simulink subsystem "MR_MainRotorForcesMoments"  (R2025a)
settings: Solver=VariableStepAuto  StartTime=0.0  StopTime=20  RelTol=1e-3
undefined symbols (not defined in the file): MR_BEDistFromEffSta_A, MR_BladeFlapInertia_P, MR_RotationMatrix_A, MR_RotorRadius_P, MR_TranslationMatrix_A
libraries: simulink_extras x4
settings Model: DataDictionary=MainRotor.sldd  EnableAccessToBaseWorkspace=off  DefaultTestHarness=MR_MainRotorForcesMoments_Harness_v1  Creator=Admin  LastModifiedBy=tunglt60

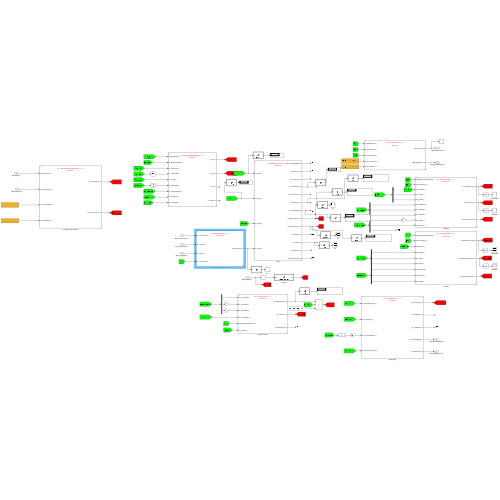
[thumbnail: Simulink's stored preview of the top-level diagram]
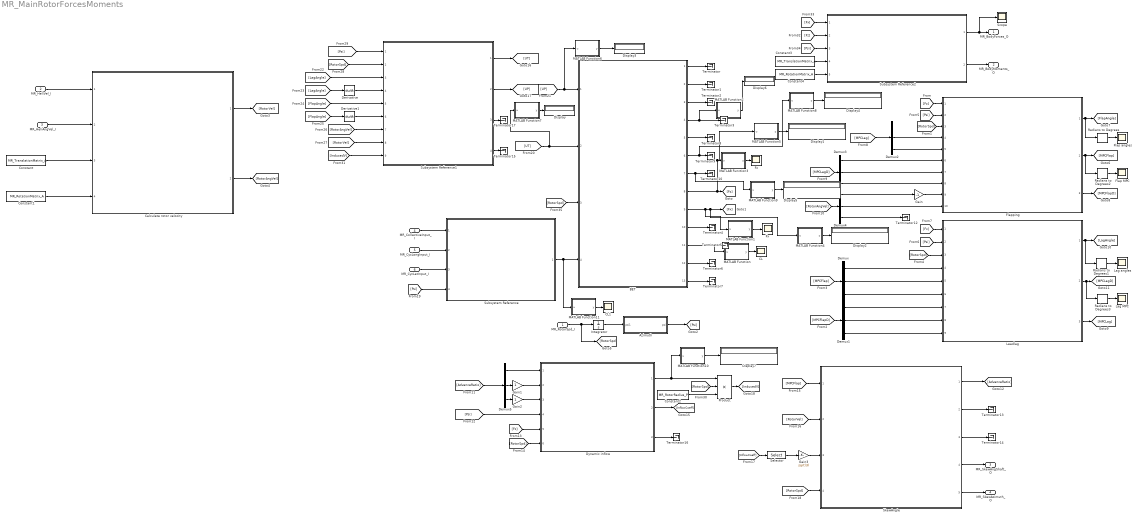
== system MR_MainRotorForcesMoments ==
  MR_RotorSpd_I : Inport
  MR_HeliVel_I : Inport  Port=2
  MR_HeliAngVel_I : Inport  Port=3
  MR_CollectiveInput_I : Inport  Port=4
  MR_CycLongInput_I : Inport  Port=5
  MR_CycLatInput_I : Inport  Port=6
  Azimuth : MATLAB Function  TreatAsAtomicUnit=on
  BET : Subsystem  ReferencedSubsystem=RT_BladeElementForces_v1_2  RT_Weight=MR_Weight_P  RT_AirDensity=MR_AirDensity_P  RT_RotorRadius=MR_RotorRadius_P  RT_NondimRadialDisRef=MR_NondimRadialDisRef_P  RT_BEDistFromEffSta=MR_BEDistFromEffSta_A  RT_SonicVel=MR_SonicVel_P  RT_SigmaAvgUH60=MR_SigmaAvgUH60_P  RT_NumberOfBlades=MR_NumberOfBlades_P  RT_TaperedRatio=MR_TaperedRatio_P
      settings: PermitHierarchicalResolution=None
  CL : Scope
      settings: ActiveDisplayYMinimum=44.632677219463247  ActiveDisplayYMaximum=47.250297558148787  DataLoggingVariableName=ScopeData5
  CL1 : Scope
      settings: ActiveDisplayYMinimum=0.59813170079773181  ActiveDisplayYMaximum=0.79813170079773177  DataLoggingVariableName=ScopeData10
  Calculate rotor velocity : Subsystem  ReferencedSubsystem=RT_HubLinearAndAngularVelocity_v1_1
      settings: PermitHierarchicalResolution=None
  Constant : Constant  Value=MR_TranslationMatrix_A
  Constant1 : Constant  Value=MR_RotationMatrix_A
  Constant2 : Constant  Value=MR_RotorRadius_P
  Constant3 : Constant  Value=MR_TranslationMatrix_A
  Constant4 : Constant  Value=MR_RotationMatrix_A
  Demux{,1..5} (6 alike) : Demux  Outputs=3
  Derivative : Derivative
  Derivative1 : Derivative
  Display{,1..7} (8 alike) : Display
  Dynamic inflow : Subsystem  ReferencedSubsystem=RT_DynamicInflow_V1_2  RT_BEDistFromEffSta=MR_BEDistFromEffSta_A  RT_AirDensity=MR_AirDensity_P  RT_RotorRadius=MR_RotorRadius_P
  Flap MPC : Scope
      settings: ActiveDisplayYMinimum=-75.476403877152109  ActiveDisplayYMaximum=118.89472721519165  DataLoggingVariableName=ScopeData4
  Flap angles : Scope
      settings: ActiveDisplayYMinimum=-1.4856198695096292  ActiveDisplayYMaximum=13.370578825586666  DataLoggingVariableName=ScopeData8
  Flapping : Subsystem  ReferencedSubsystem=RT_FlappingDynamic_v1_2  RT_BEDistFromEffSta=MR_BEDistFromEffSta_A  RT_RotorRadius=MR_RotorRadius_P  RT_BladeFlapInertia=MR_BladeFlapInertia_P*2  RT_BEMassFromHinge=MR_BEMassFromHinge_A  RT_BEDistFromHinge=MR_BEDistFromHinge_A  RT_HingeFlapPos=MR_HingeFlapPos_P
      settings: PermitHierarchicalResolution=None
  Fx : Scope
      settings: ActiveDisplayYMinimum=-148.02372012161376  ActiveDisplayYMaximum=1332.213481094524  DataLoggingVariableName=ScopeData7
  Fz : Scope
      settings: ActiveDisplayYMinimum=-361.43274494516839  ActiveDisplayYMaximum=97.915180558424424  DataLoggingVariableName=ScopeData6
  Gain : Gain  Gain=-1
  Gain1 : Gain
  Gain2 : Gain
  Gain3 : Gain  Gain=sqrt(3)
  Integrator : Integrator
  Lag MPC : Scope
      settings: ActiveDisplayYMinimum=-20550.82418968204  ActiveDisplayYMaximum=3886.6217076516573  DataLoggingVariableName=ScopeData9
  Lag angles : Scope
      settings: ActiveDisplayYMinimum=-1.032742411790134  ActiveDisplayYMaximum=9.29468170611121  DataLoggingVariableName=ScopeData3
  Leadlag : Subsystem  ReferencedSubsystem=RT_LeadLagDynamic_v1_2  RT_BEDistFromEffSta=MR_BEDistFromEffSta_A  RT_RotorRadius=MR_RotorRadius_P  RT_BEMassFrHingeLead=MR_BEMassFrHingeLead_A  RT_BEDistFrHingeLead=MR_BEDistFrHingeLead_A  RT_HingeLeadPos=MR_HingeLeadPos_P  RT_BladeLeadInertia=MR_BladeLeadInertia_P
      settings: PermitHierarchicalResolution=None
  MATLAB Function : MATLAB Function  TreatAsAtomicUnit=on
  MATLAB Function1 : MATLAB Function  TreatAsAtomicUnit=on
  MATLAB Function10 : MATLAB Function  TreatAsAtomicUnit=on
  MATLAB Function11 : MATLAB Function  TreatAsAtomicUnit=on
  MATLAB Function2 : MATLAB Function  TreatAsAtomicUnit=on
  MATLAB Function3 : MATLAB Function  TreatAsAtomicUnit=on
  MATLAB Function4 : MATLAB Function  TreatAsAtomicUnit=on
  MATLAB Function5 : MATLAB Function  TreatAsAtomicUnit=on
  MATLAB Function6 : MATLAB Function  TreatAsAtomicUnit=on
  MATLAB Function7 : MATLAB Function  TreatAsAtomicUnit=on
  MATLAB Function8 : MATLAB Function  TreatAsAtomicUnit=on
  MATLAB Function9 : MATLAB Function  TreatAsAtomicUnit=on
  Product : Product  Inputs=3
  Radians to Degrees{,1..3} (4 alike) : simulink_extras/Transformations/Radians to Degrees
  Scope : Scope
      settings: ActiveDisplayYMinimum=-141063.76400724504  ActiveDisplayYMaximum=27745.518592348737  DataLoggingVariableName=ScopeData11
  Selector : Selector  InputPortWidth=3  IndexOptions=Index vector (dialog)  Indices=1  OutputSizes=1
  SkewAngle : Subsystem  ReferencedSubsystem=RT_SkewCalculation_V1_2  RT_RotorRadius=MR_RotorRadius_P
  Subsystem Reference : Subsystem  ReferencedSubsystem=RT_BladePitchAngles_v1_2
  Subsystem Reference1 : Subsystem  ReferencedSubsystem=RT_RelativeWindOnAllBlade_v1_2  RT_BladeSegment=MR_NumberOfSegments_P  RT_BEDistFromEffSta=MR_BEDistFromEffSta_A*MR_RotorRadius_P
      settings: PermitHierarchicalResolution=None
  Subsystem Reference2 : Subsystem  ReferencedSubsystem=RT_ForcesMoments_v1_2  RT_BEDistanceToEffSta=MR_BEDistFromEffSta_A
      settings: PermitHierarchicalResolution=None
  Terminator{,1..10,12..17} (17 alike) : Terminator
  MR_BodyForces_O : Outport
  MR_BodyMoments_O : Outport  Port=2
  MR_SkewAngShaft_O : Outport  Port=3
  MR_SkewAzimuth_O : Outport  Port=4
  wires:
  BET/8 -> MATLAB Function3/1(u), MATLAB Function5/1(u), [Fz]
  BET/9 -> MATLAB Function1/1(u), [Fx], MATLAB Function4/1(u)
  BET/1 -> Terminator/1
  BET/2 -> Terminator1/1
  BET/10 -> Terminator4/1
  BET/11 -> Terminator5/1, MATLAB Function/1(u)
  BET/12 -> Terminator6/1
  BET/13 -> Terminator7/1
  BET/5 -> Terminator8/1
  BET/6 -> Terminator9/1, MATLAB Function8/1(u)
  BET/3 -> Terminator2/1
  BET/4 -> MATLAB Function2/1(u), Terminator3/1
  BET/7 -> Terminator10/1, MATLAB Function9/1(u)
  Integrator/1 -> Azimuth/1(psi1)
  Azimuth/1(psi) -> [Psi]
  MR_HeliVel_I/1 -> Calculate rotor velocity/1
  Constant/1 -> Calculate rotor velocity/3
  Constant1/1 -> Calculate rotor velocity/4
  MR_HeliAngVel_I/1 -> Calculate rotor velocity/2
  Calculate rotor velocity/2 -> [RotorAngVel]
  Calculate rotor velocity/1 -> [RotorVel]
  [Fz] -> Flapping/1
  MR_RotorSpd_I/1 -> [RotorSpd], Integrator/1
  [RotorSpd] -> Flapping/3
  Flapping/3 -> [MPCFlapD]
  Flapping/1 -> Radians to Degrees/1, [FlapAngle]
  Leadlag/1 -> Radians to Degrees1/1, [LagAngle]
  Leadlag/2 -> [MPCLagD], Radians to Degrees3/1
  Leadlag/3 -> [MPCLag]
  Demux/1 -> Leadlag/4
  Demux/2 -> Leadlag/5
  Demux/3 -> Leadlag/6
  [MPCFlap] -> Demux/1
  [MPCFlapD] -> Demux1/1
  Demux1/2 -> Leadlag/8
  Demux1/1 -> Leadlag/7
  Demux1/3 -> Leadlag/9
  [RotorSpd] -> Leadlag/3
  [Psi] -> Flapping/2
  [Psi] -> Leadlag/2
  [Fx] -> Leadlag/1
  [MPCLag] -> Demux2/1
  [MPCLagD] -> Demux3/1
  Demux3/1 -> Flapping/6
  [RotorAngVel] -> Demux4/1
  Demux4/1 -> Gain/1
  Gain/1 -> Flapping/9
  Demux4/2 -> Flapping/10
  Demux4/3 -> Terminator12/1
  Demux3/2 -> Flapping/7
  Demux3/3 -> Flapping/8
  Gain1/1 -> Dynamic inflow/2
  Gain2/1 -> Dynamic inflow/3
  SkewAngle/1 -> [AdvanceRatio]
  SkewAngle/2 -> Terminator13/1
  SkewAngle/3 -> Terminator14/1
  SkewAngle/4 -> MR_SkewAngShaft_O/1
  SkewAngle/5 -> MR_SkewAzimuth_O/1
  Demux5/2 -> Gain1/1
  Demux5/3 -> Gain2/1
  Demux5/1 -> Dynamic inflow/1
  [AdvanceRatio] -> Demux5/1
  [Psi] -> Dynamic inflow/4
  [Fz] -> Dynamic inflow/5
  [RotorSpd] -> Dynamic inflow/6
  [MPCFlap] -> SkewAngle/1
  [RotorVel] -> SkewAngle/2
  Dynamic inflow/2 -> [InflowCoeff]
  Dynamic inflow/3 -> Terminator16/1
  [InflowCoeff] -> Selector/1
  Selector/1 -> Gain3/1
  Gain3/1 -> SkewAngle/3
  [RotorSpd] -> SkewAngle/4
  MR_CycLongInput_I/1 -> Subsystem Reference/2
  MR_CycLatInput_I/1 -> Subsystem Reference/3
  MR_CollectiveInput_I/1 -> Subsystem Reference/1
  [Psi] -> Subsystem Reference/4
  Subsystem Reference/1 -> BET/4, MATLAB Function11/1(u)
  Subsystem Reference1/4 -> Terminator15/1
  Subsystem Reference1/2 -> [UP]
  Subsystem Reference1/1 -> [UT]
  [UT] -> MATLAB Function7/1(u), BET/2
  [UP] -> BET/1, MATLAB Function6/1(u)
  [RotorAngVel] -> Subsystem Reference1/7
  [RotorVel] -> Subsystem Reference1/8
  [RotorSpd] -> Subsystem Reference1/2
  [Psi] -> Subsystem Reference1/1
  Dynamic inflow/1 -> Product/1, MATLAB Function10/1(u)
  Constant2/1 -> Product/3
  [RotorSpd] -> Product/2
  Product/1 -> [InducedV]
  [InducedV] -> Subsystem Reference1/9
  Subsystem Reference1/3 -> Terminator17/1
  [Fz] -> Subsystem Reference2/2
  [Fx] -> Subsystem Reference2/1
  [Psi] -> Subsystem Reference2/3
  Constant4/1 -> Subsystem Reference2/5
  Constant3/1 -> Subsystem Reference2/4
  Subsystem Reference2/2 -> MR_BodyMoments_O/1
  Subsystem Reference2/1 -> MR_BodyForces_O/1, Scope/1
  [RotorSpd] -> BET/3
  Radians to Degrees/1 -> Flap angles/1
  Radians to Degrees1/1 -> Lag angles/1
  Radians to Degrees2/1 -> Flap MPC/1
  Flapping/2 -> [MPCFlap], Radians to Degrees2/1
  Radians to Degrees3/1 -> Lag MPC/1
  [LagAngle] -> Derivative/1
  [FlapAngle] -> Derivative1/1
  [LagAngle] -> Subsystem Reference1/3
  Derivative/1 -> Subsystem Reference1/4
  [FlapAngle] -> Subsystem Reference1/5
  Derivative1/1 -> Subsystem Reference1/6
  MATLAB Function/1(y) -> CL/1
  MATLAB Function1/1(y) -> Fx/1
  MATLAB Function2/1(y) -> Display6/1
  MATLAB Function3/1(y) -> Fz/1
  Demux2/2 -> Flapping/4
  Demux2/3 -> Flapping/5
  MATLAB Function4/1(y) -> Display2/1
  MATLAB Function5/1(y) -> Display1/1
  MATLAB Function6/1(y) -> Display3/1
  MATLAB Function7/1(y) -> Display/1
  MATLAB Function8/1(y) -> Display4/1
  MATLAB Function9/1(y) -> Display5/1
  MATLAB Function10/1(y) -> Display7/1
  MATLAB Function11/1(y) -> CL1/1

== matlab function MR_MainRotorForcesMoments/MATLAB Function ==
  data: u input; y output
function y = extract(u)

y = [u(1,1);u(1,20)];

== matlab function MR_MainRotorForcesMoments/MATLAB Function1 ==
  data: u input; y output
function y = extract(u)

y = [u(1,1);u(1,20)];

== matlab function MR_MainRotorForcesMoments/MATLAB Function2 ==
  data: u input; y output
function y = extract(u)

y = [u(1,1);u(1,20)];

== matlab function MR_MainRotorForcesMoments/MATLAB Function3 ==
  data: u input; y output
function y = extract(u)

y = [u(1,1);u(1,20)];

== matlab function MR_MainRotorForcesMoments/MATLAB Function4 ==
  data: u input; y output
function y = sum(u)

y = sum(u,2);

== matlab function MR_MainRotorForcesMoments/MATLAB Function5 ==
  data: u input; y output
function y = sum(u)

y = sum(u,2);

== matlab function MR_MainRotorForcesMoments/MATLAB Function6 ==
  data: u input; y output
function y = extract(u)

y = [u(1,1);u(1,20)];

== matlab function MR_MainRotorForcesMoments/MATLAB Function7 ==
  data: u input; y output
function y = extract(u)

y = [u(1,1);u(1,20)];

== matlab function MR_MainRotorForcesMoments/Azimuth ==
  data: psi1 input; psi output
function psi = AzimuthCalculation(psi1)

psi = [psi1;psi1+pi/2;psi1+pi;psi1+3*pi/2];
psi = mod(psi,2*pi);

== matlab function MR_MainRotorForcesMoments/MATLAB Function8 ==
  data: u input; y output
function y = sum(u)

y = sum(u,2);

== matlab function MR_MainRotorForcesMoments/MATLAB Function9 ==
  data: u input; y output
function y = sum(u)

y = sum(u,2);

== matlab function MR_MainRotorForcesMoments/MATLAB Function10 ==
  data: u input; y output
function y = extract(u)

y = [u(1,1);u(1,20)];

== matlab function MR_MainRotorForcesMoments/MATLAB Function11 ==
  data: u input; y output
function y = extract(u)

y = [u(1,1);u(1,20)];
